simulink model "Smoothing"  (Simulink 7.0)
settings: Solver=ode45  StartTime=0.0  StopTime=10.0  RelTol=1e-3
settings Model: Creator=volgy  LastModifiedBy=volgy

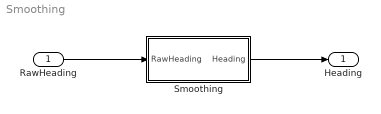
== system Smoothing ==
  RawHeading : Inport  OutDataType=sfix(16)  OutScaling=2^0
  Smoothing : Subsystem
  Heading : Outport  OutDataType=sfix(16)  OutScaling=2^0
  wires:
  RawHeading/1 -> Smoothing/1(RawHeading)
  Smoothing/1(Heading) -> Heading/1

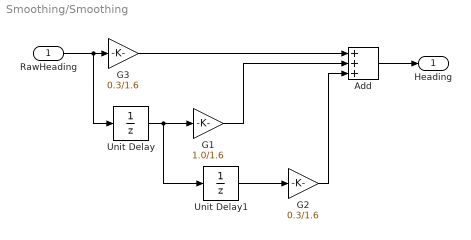
== system Smoothing/Smoothing ==
  RawHeading : Inport  OutDataType=sfix(16)  OutScaling=2^0
  Add : Sum  Inputs=+++  OutDataType=sfix(16)  OutScaling=2^-10
  G1 : Gain  Gain=1.0/1.6  ParameterDataType=sfix(16)  ParameterScaling=2^0  OutDataType=sfix(16)  OutScaling=2^0
  G2 : Gain  Gain=0.3/1.6  ParameterDataType=sfix(16)  ParameterScaling=2^0  OutDataType=sfix(16)  OutScaling=2^0
  G3 : Gain  Gain=0.3/1.6  ParameterDataType=sfix(16)  ParameterScaling=2^0  OutDataType=sfix(16)  OutScaling=2^0
  Unit Delay : UnitDelay
  Unit Delay1 : UnitDelay  SampleTime=-1
  Heading : Outport  OutDataType=sfix(16)  OutScaling=2^0
  wires:
  Add/1 -> Heading/1
  G2/1 -> Add/3
  Unit Delay1/1 -> G2/1
  G1/1 -> Add/2
  Unit Delay/1 -> Unit Delay1/1, G1/1
  G3/1 -> Add/1
  RawHeading/1 -> Unit Delay/1, G3/1
